simulink model "transformer_saturation"  (R2014a)
settings: Solver=ode23tb  StartTime=0.0  StopTime=1/20  MaxStep=1e-4  RelTol=1e-4
undefined symbols (not defined in the file or in its folder): D1, Delta
libraries: powerlib x12, simulink x1
settings Model: Creator=cosorio  LastModifiedBy=cosorio
settings DebuggingCC: UnconnectedInputMsg=none  UnconnectedOutputMsg=none  UnconnectedLineMsg=none

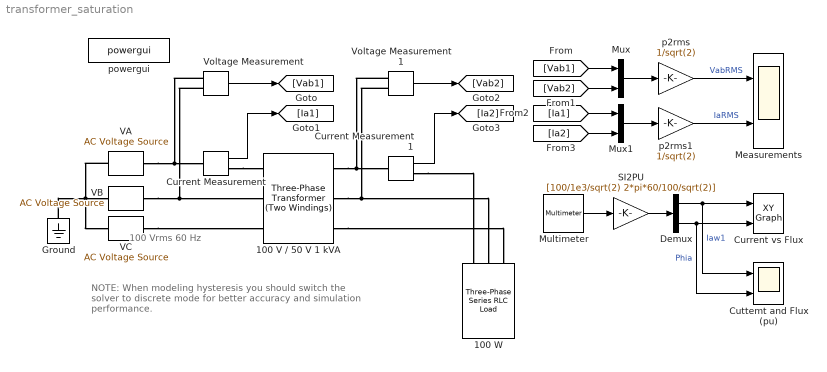
== system transformer_saturation ==
  note: 100 Vrms
      | 60 Hz
  note: NOTE:
      | When modeling hysteresis you should switch
      | the solver to discrete mode for better accuracy
      | and simulation performance.
  100 V / 50 V 1 kVA : powerlib/Elements/Three-Phase Transformer (Two Windings)  Winding1Connection=Yg  UNITS=pu  NominalPower=[ 1e3 , 60 ]  Winding1=[ 100 , 0.002 , 1e-3]  Winding2Connection=Delta (D1)  Winding2=[ 50 , 0.002 , 1e-3]  SetSaturation=on  Rm=5000  Lm=5000  Saturation=[ 0, 0 ; 0.001, 0.5 ; 1, 0.8 ]  Hysteresis=off  DataFile='myhysteresis'  SetInitialFlux=off  InitialFluxes=[-0.999799660126556 0.499986536618418 0.499813123666584]  Measurements=All measurements (V I Fluxes)  MoreParameters=off  BreakLoop=on  DataType=off  TransfoNumber=1
  100 W : powerlib/Elements/Three-Phase Series RLC Load  LConnTagsString=A|B|C  Configuration=Y (grounded)  NominalVoltage=50  NominalFrequency=60  ActivePower=100  InductivePower=0  CapacitivePower=0  Measurements=None  LoadType=constant Z
  Current Measurement : powerlib/Measurements/Current Measurement  PhasorSimulation=off  OutputType=Complex  PSBequivalent=0
  Current Measurement1 : powerlib/Measurements/Current Measurement  PhasorSimulation=off  OutputType=Complex  PSBequivalent=0
  Current vs Flux : simulink/Sinks/XY Graph  xmin=-1  xmax=1  ymin=-1  ymax=1  st=-1
  Cuttemt and Flux (pu) : Scope  NumInputPorts=2
      settings: YMin=-1~-1  YMax=1~1
  Demux : Demux  Outputs=2
  Ground : powerlib/Elements/Ground  LConnTagsString=a
  Measurements : Scope  NumInputPorts=2
      settings: YMin=-150~-10  YMax=150~10
  Multimeter : powerlib/Measurements/Multimeter  PhasorSimulation=off  OutputType=Complex  sel=[7 19]  L=21  Gain=[1 1]  yselected={'Iag_w1: 100 V // 50 V 1 kVA','Flux_A: 100 V // 50 V 1 kVA'};  PSBOutputType=1  PSBequivalent=0  AxesSetting=[0,0.1,-100,100]  Display=0  SavedBlockNames=-11
  Mux : Mux  Inputs=2
  Mux1 : Mux  Inputs=2
  SI2PU : Gain  Gain=[100/1e3/sqrt(2) 2*pi*60/100/sqrt(2)]
  VA : powerlib/Electrical Sources/AC Voltage Source  Amplitude=100*sqrt(2)/sqrt(3)  Phase=0  Frequency=60  SampleTime=0  Measurements=None
  VB : powerlib/Electrical Sources/AC Voltage Source  Amplitude=100*sqrt(2)/sqrt(3)  Phase=-120  Frequency=60  SampleTime=0  Measurements=None
  VC : powerlib/Electrical Sources/AC Voltage Source  Amplitude=100*sqrt(2)/sqrt(3)  Phase=120  Frequency=60  SampleTime=0  Measurements=None
  Voltage Measurement : powerlib/Measurements/Voltage Measurement  PhasorSimulation=off  OutputType=Complex  PSBequivalent=0
  Voltage Measurement1 : powerlib/Measurements/Voltage Measurement  PhasorSimulation=off  OutputType=Complex  PSBequivalent=0
  p2rms : Gain  Gain=1/sqrt(2)
  p2rms1 : Gain  Gain=1/sqrt(2)
  powergui : powerlib/powergui  Priority=1  SimulationMode=Continuous  SolverType=Tustin  SampleTime=5e-6  frequency=60  SPID=off  DisableSnubberDevices=off  DisableRonSwitches=off  DisableVfSwitches=off  SwTol=0  Interpol=off  DisplayEquations=off  Ts=0  methode=off  frequencyindice=60  Pbase=100e6  ErrMax=1e-4  Iterations=50  UnitsV=kV  UnitsW=MW  FunctionMessages=off  echomessages=off  HookPort=off  EnableUseOfTLC=off  x0status=blocks  RestoreLinks=warning  ResistiveCurrentMeasurement=off  Frange=[0:2:500]  Ylog=off  Xlog=on  ShowGrid=off  save=off  variable=ZData  structure=0  ZoomFFT=off  StartTime=0.0  cycles=1  DisplayStyle=1  fundamental=60  FreqAxis=off  MaxFrequency=1000  frequencyindicesteady=1  RmsSteady=1  display=off
  wires:
  Voltage Measurement/1 -> [Vab1]
  Current Measurement/1 -> [Ia1]
  Voltage Measurement1/1 -> [Vab2]
  Current Measurement1/1 -> [Ia2]
  [Vab1] -> Mux/1
  [Ia2] -> Mux1/2
  [Ia1] -> Mux1/1
  [Vab2] -> Mux/2
  p2rms/1 -> Measurements/1  "VabRMS"
  Mux/1 -> p2rms/1
  Mux1/1 -> p2rms1/1
  Multimeter/1 -> SI2PU/1
  Demux/1 -> Cuttemt and Flux (pu)/1, Current vs Flux/1  "Iaw1"
  Demux/2 -> Cuttemt and Flux (pu)/2, Current vs Flux/2  "Phia"
  p2rms1/1 -> Measurements/2  "IaRMS"
  SI2PU/1 -> Demux/1
  connections:
  VA/LConn1 -- Ground/LConn1 -- VC/LConn1 -- VB/LConn1
  VB/RConn1 -- 100 V / 50 V 1 kVA/LConn2 -- Voltage Measurement/LConn2
  VC/RConn1 -- 100 V / 50 V 1 kVA/LConn3
  100 V / 50 V 1 kVA/RConn3 -- 100 W/LConn3
  100 V / 50 V 1 kVA/RConn2 -- 100 W/LConn2 -- Voltage Measurement1/LConn2
  VA/RConn1 -- Current Measurement/LConn1 -- Voltage Measurement/LConn1
  Current Measurement/RConn1 -- 100 V / 50 V 1 kVA/LConn1
  100 V / 50 V 1 kVA/RConn1 -- Current Measurement1/LConn1 -- Voltage Measurement1/LConn1
  Current Measurement1/RConn1 -- 100 W/LConn1
